simulink model "HIL_Testing_SW"  (Simulink 7.5)
settings: Solver=ode1  StartTime=0.0  StopTime=Inf  FixedStep=0.001  RelTol=1e-3
PostLoadFcn:
  | , if any(exist('dsrtsu_mdlpostloadfcn', 'file') == [2, 3, 6]), try dsrtsu_mdlpostloadfcn('Execute', bdroot); catch fprintf('Error in PostLoadFcn (dsrtsu_mdlpostloadfcn) for model "%s":\n %s\n', bdroot, lasterr); end, end,
undefined symbols (not defined in the file): CeBSER_Cnt_NumTempAxisPts, ChargeCord, ChargeCord_Control, ChargeToSOCCurr, ChrgCurrLim, CrntSens1Fine, CS_SOCSetPt, CyclerMaxChrgPwr, CyclerMaxDschrgPwr, deltaAhr, Drive_1, Drive_10, Drive_11, Drive_12, Drive_13, Drive_14, Drive_15, Drive_16, Drive_17, Drive_18, Drive_19, Drive_2, Drive_20, Drive_21, Drive_22, Drive_23, Drive_24, Drive_25, Drive_26, Drive_27, Drive_28, Drive_29, Drive_3, Drive_30, Drive_31, Drive_32, Drive_33, Drive_34, Drive_35, Drive_36, Drive_37, Drive_38, Drive_39, Drive_4, Drive_40, Drive_41, Drive_42, Drive_43, Drive_44, Drive_45, Drive_46, Drive_47, Drive_48, Drive_49, Drive_5, Drive_50, Drive_51, Drive_6, Drive_7, Drive_8 ... (+50)
libraries: simulink x129, rtican x50, rti2211sailib x5, rti2211serlib x5, rti2202miolib x3
(part 10 of 23)

== system HIL_Testing_SW/RX/Read EREV/Read PTEX ==
  Constant : Constant  Value=-1  OutDataType=fixdt(1, 16)  OutScaling=2^0
  PPEI_High_Vlt_Battery_Vlt_Status1 : rtican/RTICAN Receive (RX)   SystemSampleTime=-1  Reserved1=[]  Reserved2=[]  Reserved3=[]  Reserved4=[]  SfcnMessage=[]  Msg_Struct=[]  BoardTypeNo=[]  BoardNo=[]  ChannelNo=[]  Parameters=[]  DialogFcn=[]  UnitName=[]  Revision=[]  UnitValues=[]  DSProperties=struct('RTI',struct('Version',uint32(5),'BlockType',struct('isSLSource',uint8(1),'isSLSink',uint8(1),'isHWSource',uint8(0),'isHWSink',uint8(0),'isSetup',uint8(0),'isInline',uint8(1),'isNonInline',uint8(0),'isInterrupt',uint8(0),'isChannelwise',uint8(0)),'IOBoardType','RTICAN','UnitType','MESSAGE','Identifier','RX','DialogType','MSVC','BlockSet','RTICAN','SlaveProcessor','CAN'))  RTIBlockInterface=struct('OutputPortsWidth',int32([1 1 1 1 1 1 1 1]),'OutputPortsActive',[1 1 1 1 1 1 1 1],'OutputPortsName',{{'HVBatVltLwLmtCrnk','HVBatVltLwLmtCrnkV','HVBatVltLwLmt','HVBatVltLwLmtV','HVBatVltUpLmt','HVBatVltUpLmtV','HVBatPackPrcdVltg','HVBatPackPrcdVltgV'}},'OutputPortsDataType',{{'SS_DOUBLE','SS_DOUBLE','SS_DOUBLE','SS_DOUBLE','SS_DOUBLE','SS_DOUBLE','SS_DOUBLE','SS_DOUBLE'}},'OutputPortsLabel',{{'HVBatVltLwLmtCrnk','HVBatVltLwLmtCrnkV','HVBatVltLwLmt','HVBatVltLwLmtV','HVBatVltUpLmt','HVBatVltUpLmtV','HVBatPackPrcdVltg','HVBatPackPrcdVltgV'}},'OutputPortsLabelMode','ON','InputPortsWidth',int32(0),'InputPortsActive',0,'DialogFcn','rtican_message_interface_gui','BlockDisplay',{{'','center'}},'IconTransparency','on','ParameterTunableNames',{{}},'InitLevel',3,'BlockName',struct('Token',{{'PPEI_High_Vlt_Battery_Vlt_Status'}}),'SampleTime',{{-1}},'TriggerPort',{{'none'}},'EnablePort',{{'none'}})  RTIBlockParameters=struct('BoardTypeNo',{{4302,'OFF',[]}},'BoardNo',{{1,'ON',[1 16]}},'ChannelNo',{{2,'ON',[1 4]}},'Parameters',{{struct('DataFileSupport',struct('DataFileSelectedMaster',1,'DataFileSelectedLocal',1,'DataFileName',['c:\data\databases\8.4.5 (140425)\globala - pe.dbc|'],'DataFileDate',{{{['24-Apr-2014 15:33:48']}}},'SelectedFile',['..\databases\8.4.5 (140425)\globala - pe.dbc'],'InterfaceFcn','rtican_dbc_file_parser'),'Options',struct('StatusSelected',0,'TimeSelected',0,'DeltaTimeSelected',0,'BytePortSelected',0,'MessageLengthSelected',0,'TriggerPort',struct('Selected',0,'TriggerType',0),'UserCoding',struct('Selected',0,'InterfaceFile','UserDecodingFile','FcnName','UserDecodeFcn','InportSelected',0,'InportWidth',1,'OutportSelected',0,'OutportWidth',1),'EnablePortSelected',0,'SignalOnPortnameSelected',1,'UseRXService',0),'Message',struct('MsgOnBlocknameSelected',1,'MsgName','PPEI_High_Vlt_Battery_Vlt_Status','MsgIdFormat',0,'MsgId',983,'MsgLength',8,'NumSignals',8,'SampleTime',-1,'Signal',struct('SgnName',{'HVBatVltLwLmtCrnk','HVBatVltLwLmtCrnkV','HVBatVltLwLmt','HVBatVltLwLmtV','HVBatVltUpLmt','HVBatVltUpLmtV','HVBatPackPrcdVltg','HVBatPackPrcdVltgV'},'SgnStartBit',{0,10,16,26,32,42,48,58},'SgnLength',{10,1,10,1,10,1,10,1},'SgnType',{0,0,0,0,0,0,0,0},'ModeValue',{-1,-1,-1,-1,-1,-1,-1,-1},'DataType',{0,0,0,0,0,0,0,0},'ByteLayout',{2,2,2,2,2,2,2,2},'Factor',{0.52,1,0.52,1,0.52,1,0.52,1},'Offset',{0,0,0,0,0,0,0,0},'SgnComment',{{''},{''},{''},{''},{''},{''},{''},{''}},'SgnUnit',{'V','','V','','V','','V',''},'Min',{0,0,0,0,0,0,0,0},'Max',{531.96,1,531.96,1,531.96,1,531.96,1},'SLDataType',{'SS_DOUBLE','SS_DOUBLE','SS_DOUBLE','SS_DOUBLE','SS_DOUBLE','SS_DOUBLE','SS_DOUBLE','SS_DOUBLE'}),'MsgIdNumFormat',0,'MsgComment',{{''}}),'Version',1.2,'general',struct('isFromLib',0)),'OFF',[]}},'GroupId',{{struct('Group',{{'RTICAN'}},'No',5,'Behavior',{{'NAMECHANGE'}},'BlockType',{{'SINK'}},'NameChangeFlag',0),'OFF',[]}},'SFcnRTICANMessage',{{struct('MsgType','RX','SFcnPortType','Scalar','MsgName','PPEI_High_Vlt_Battery_Vlt_Status','MsgIdFormat','STD','MsgId',983,'MsgLength',8,'NumSignals',8,'SampleTime',-1,'Signal',struct('SgnName',{'HVBatVltLwLmtCrnk','HVBatVltLwLmtCrnkV','HVBatVltLwLmt','HVBatVltLwLmtV','HVBatVltUpLmt','HVBatVltUpLmtV','HVBatPackPrcdVltg','HVBatPackPrcdVltgV'},'SgnStartBit',{0,10,16,26,32,42,48,58},'SgnLength',{10,1,10,1,10,1,10,1},'SgnType',{'standard','standard','standard','standard','standard','standard','standard','standard'},'ModeValue',{-1,-1,-1,-1,-1,-1,-1,-1},'DataType',{['unsigned int'],['unsigned int'],['unsigned int'],['unsigned int'],['unsigned int'],['unsigned int'],['unsigned int'],['unsigned int']},'ByteLayout',{['motorola back.'],['motorola back.'],['motorola back.'],['motorola back.'],['motorola back.'],['motorola back.'],['motorola back.'],['motorola back.']},'Factor',{0.52,1,0.52,1,0.52,1,0.52,1},'Offset',{0,0,0,0,0,0,0,0},'SLDataType',{'SS_DOUBLE','SS_DOUBLE','SS_DOUBLE','SS_DOUBLE','SS_DOUBLE','SS_DOUBLE','SS_DOUBLE','SS_DOUBLE'}),'StatusSelected','no','TimeSelected','no','DeltaTimeSelected','no','BytePortSelected','no','MessageLengthSelected','no','TriggerPort',struct('Selected','no','TriggerType',0),'UserCoding',struct('Selected','no','InterfaceFile','UserDecodingFile','FcnName','UserDecodeFcn','InportSelected','no','InportWidth',1,'OutportSelected','no','OutportWidth',1),'EnablePortSelected','no','UseRXService','no','BoardType','DS4302','BoardNo',1,'ControllerNo',2),'OFF',[]}},'TLCFileName',{{'rtican_rx_message','OFF',[]}})  RTISFcnParameters=struct('SFcnRTICANMessage','struct','TLCFileName','char')  RTIBlockParaDefault=struct('BoardTypeNo',4302,'BoardNo',1,'ChannelNo',1,'Parameters',struct('DataFileSupport',struct('DataFileSelectedMaster',0,'DataFileSelectedLocal',0,'DataFileName','','DataFileDate','','SelectedFile',['<no file selected>']),'Options',struct('StatusSelected',1,'TimeSelected',1,'DeltaTimeSelected',1,'BytePortSelected',0,'MessageLengthSelected',0,'TriggerPort',struct('Selected',0,'TriggerType','rising'),'UserCoding',struct('Selected',0,'InterfaceFile','UserDecodingFile','FcnName','UserDecodeFcn','InportSelected',0,'InportWidth',1,'OutportSelected',0,'OutportWidth',1),'EnablePortSelected',0,'SignalOnPortnameSelected',1,'UseRXService',0),'Message',struct('MsgOnBlocknameSelected',0,'MsgName',['RX Message'],'MsgIdFormat',0,'MsgId',100,'MsgLength',8,'NumSignals',1,'SampleTime',-1,'Signal',struct('SgnName',['RX signal'],'SgnStartBit',0,'SgnLength',8,'SgnType',0,'ModeValue',-1,'DataType',0,'SLDataType','SS_DOUBLE','ByteLayout',0,'Factor',1,'Offset',0,'Min',0,'Max',255,'SgnComment',{{}},'SgnUnit',''),'MsgIdNumFormat',0,'MsgComment',{{''}}),'Version',1.2,'general',struct('isFromLib',1)),'GroupId',struct('Group',{{'RTICAN'}},'No',1,'Behavior',{{'NAMECHANGE'}},'BlockType',{{'SINK'}},'NameChangeFlag',0),'SFcnRTICANMessage',struct('MsgType','RX','MsgName',['RX Message'],'MsgIdFormat','STD','MsgId',100,'MsgLength',8,'NumSignals',1,'SampleTime',-1,'Signal',struct('SgnName',['RX signal'],'SgnStartBit',0,'SgnLength',8,'SgnType','standard','ModeValue',-1,'DataType',['unsigned int'],'ByteLayout',['little endian'],'SLDataType','SS_DOUBLE','Factor',1,'Offset',0),'StatusSelected','yes','TimeSelected','yes','DeltaTimeSelected','yes','BytePortSelected','no','MessageLengthSelected','no','EnablePortSelected','no','UserCoding',struct('Selected','no','InterfaceFile','UserDecodingFile','FcnName','UserDecodeFcn','InportSelected','no','InportWidth',1,'OutportSelected','no','OutportWidth',1),'TriggerPort',struct('Selected','no','TriggerType','rising'),'UseRXService','no','BoardType','DS4302','BoardNo',1,'ControllerNo',1,'SFcnPortType','Scalar'),'TLCFileName','rtican_rx_message')
      settings: AttributesFormatString=Group Id: RTICAN5\n
  PPEI_High_Volt_Batt_Current_Stat : rtican/RTICAN Receive (RX)   SystemSampleTime=-1  Reserved1=[]  Reserved2=[]  Reserved3=[]  Reserved4=[]  SfcnMessage=[]  Msg_Struct=[]  BoardTypeNo=[]  BoardNo=[]  ChannelNo=[]  Parameters=[]  DialogFcn=[]  UnitName=[]  Revision=[]  UnitValues=[]  DSProperties=struct('RTI',struct('Version',uint32(5),'BlockType',struct('isSLSource',uint8(1),'isSLSink',uint8(1),'isHWSource',uint8(0),'isHWSink',uint8(0),'isSetup',uint8(0),'isInline',uint8(1),'isNonInline',uint8(0),'isInterrupt',uint8(0),'isChannelwise',uint8(0)),'IOBoardType','RTICAN','UnitType','MESSAGE','Identifier','RX','DialogType','MSVC','BlockSet','RTICAN','SlaveProcessor','CAN'))  RTIBlockInterface=struct('OutputPortsWidth',int32([1 1 1 1 1 1]),'OutputPortsActive',[1 1 1 1 1 1],'OutputPortsName',{{'HVBatStOfChrgMin','HVBatCrntLwLmt','HVBatCrntLwLmtV','HVBatCrntUpLmt','HVBatCrntUpLmtV','HVBatSOCTrgtHiRes'}},'OutputPortsDataType',{{'SS_DOUBLE','SS_DOUBLE','SS_DOUBLE','SS_DOUBLE','SS_DOUBLE','SS_DOUBLE'}},'OutputPortsLabel',{{'HVBatStOfChrgMin','HVBatCrntLwLmt','HVBatCrntLwLmtV','HVBatCrntUpLmt','HVBatCrntUpLmtV','HVBatSOCTrgtHiRes'}},'OutputPortsLabelMode','ON','InputPortsWidth',int32(0),'InputPortsActive',0,'DialogFcn','rtican_message_interface_gui','BlockDisplay',{{'','center'}},'IconTransparency','on','ParameterTunableNames',{{}},'InitLevel',3,'BlockName',struct('Token',{{'PPEI_High_Volt_Batt_Current_Stat'}}),'SampleTime',{{-1}},'TriggerPort',{{'none'}},'EnablePort',{{'none'}})  RTIBlockParameters=struct('BoardTypeNo',{{4302,'OFF',[]}},'BoardNo',{{1,'ON',[1 16]}},'ChannelNo',{{2,'ON',[1 4]}},'Parameters',{{struct('DataFileSupport',struct('DataFileSelectedMaster',1,'DataFileSelectedLocal',1,'DataFileName',['c:\data\databases\8.4.5 (140425)\globala - pe.dbc|'],'DataFileDate',{{{['24-Apr-2014 15:33:48']}}},'SelectedFile',['..\databases\8.4.5 (140425)\globala - pe.dbc'],'InterfaceFcn','rtican_dbc_file_parser'),'Options',struct('StatusSelected',0,'TimeSelected',0,'DeltaTimeSelected',0,'BytePortSelected',0,'MessageLengthSelected',0,'TriggerPort',struct('Selected',0,'TriggerType',0),'UserCoding',struct('Selected',0,'InterfaceFile','UserDecodingFile','FcnName','UserDecodeFcn','InportSelected',0,'InportWidth',1,'OutportSelected',0,'OutportWidth',1),'EnablePortSelected',0,'SignalOnPortnameSelected',1,'UseRXService',0),'Message',struct('MsgOnBlocknameSelected',1,'MsgName','PPEI_High_Volt_Batt_Current_Stat','MsgIdFormat',0,'MsgId',981,'MsgLength',8,'NumSignals',6,'SampleTime',-1,'Signal',struct('SgnName',{'HVBatStOfChrgMin','HVBatCrntLwLmt','HVBatCrntLwLmtV','HVBatCrntUpLmt','HVBatCrntUpLmtV','HVBatSOCTrgtHiRes'},'SgnStartBit',{0,16,27,32,43,48},'SgnLength',{8,11,1,11,1,16},'SgnType',{0,0,0,0,0,0},'ModeValue',{-1,-1,-1,-1,-1,-1},'DataType',{0,0,0,0,0,0},'ByteLayout',{2,2,2,2,2,2},'Factor',{0.392157,0.3,1,0.3,1,0.001526},'Offset',{0,0,0,0,0,0},'SgnComment',{{''},{''},{''},{''},{''},{''}},'SgnUnit',{'','A','','A','','%'},'Min',{0,0,0,0,0,0},'Max',{100.000035,614.1,1,614.1,1,100},'SLDataType',{'SS_DOUBLE','SS_DOUBLE','SS_DOUBLE','SS_DOUBLE','SS_DOUBLE','SS_DOUBLE'}),'MsgIdNumFormat',0,'MsgComment',{{''}}),'Version',1.2,'general',struct('isFromLib',0)),'OFF',[]}},'GroupId',{{struct('Group',{{'RTICAN'}},'No',5,'Behavior',{{'NAMECHANGE'}},'BlockType',{{'SINK'}},'NameChangeFlag',0),'OFF',[]}},'SFcnRTICANMessage',{{struct('MsgType','RX','SFcnPortType','Scalar','MsgName','PPEI_High_Volt_Batt_Current_Stat','MsgIdFormat','STD','MsgId',981,'MsgLength',8,'NumSignals',6,'SampleTime',-1,'Signal',struct('SgnName',{'HVBatStOfChrgMin','HVBatCrntLwLmt','HVBatCrntLwLmtV','HVBatCrntUpLmt','HVBatCrntUpLmtV','HVBatSOCTrgtHiRes'},'SgnStartBit',{0,16,27,32,43,48},'SgnLength',{8,11,1,11,1,16},'SgnType',{'standard','standard','standard','standard','standard','standard'},'ModeValue',{-1,-1,-1,-1,-1,-1},'DataType',{['unsigned int'],['unsigned int'],['unsigned int'],['unsigned int'],['unsigned int'],['unsigned int']},'ByteLayout',{['motorola back.'],['motorola back.'],['motorola back.'],['motorola back.'],['motorola back.'],['motorola back.']},'Factor',{0.392157,0.3,1,0.3,1,0.001526},'Offset',{0,0,0,0,0,0},'SLDataType',{'SS_DOUBLE','SS_DOUBLE','SS_DOUBLE','SS_DOUBLE','SS_DOUBLE','SS_DOUBLE'}),'StatusSelected','no','TimeSelected','no','DeltaTimeSelected','no','BytePortSelected','no','MessageLengthSelected','no','TriggerPort',struct('Selected','no','TriggerType',0),'UserCoding',struct('Selected','no','InterfaceFile','UserDecodingFile','FcnName','UserDecodeFcn','InportSelected','no','InportWidth',1,'OutportSelected','no','OutportWidth',1),'EnablePortSelected','no','UseRXService','no','BoardType','DS4302','BoardNo',1,'ControllerNo',2),'OFF',[]}},'TLCFileName',{{'rtican_rx_message','OFF',[]}})  RTISFcnParameters=struct('SFcnRTICANMessage','struct','TLCFileName','char')  RTIBlockParaDefault=struct('BoardTypeNo',4302,'BoardNo',1,'ChannelNo',1,'Parameters',struct('DataFileSupport',struct('DataFileSelectedMaster',0,'DataFileSelectedLocal',0,'DataFileName','','DataFileDate','','SelectedFile',['<no file selected>']),'Options',struct('StatusSelected',1,'TimeSelected',1,'DeltaTimeSelected',1,'BytePortSelected',0,'MessageLengthSelected',0,'TriggerPort',struct('Selected',0,'TriggerType','rising'),'UserCoding',struct('Selected',0,'InterfaceFile','UserDecodingFile','FcnName','UserDecodeFcn','InportSelected',0,'InportWidth',1,'OutportSelected',0,'OutportWidth',1),'EnablePortSelected',0,'SignalOnPortnameSelected',1,'UseRXService',0),'Message',struct('MsgOnBlocknameSelected',0,'MsgName',['RX Message'],'MsgIdFormat',0,'MsgId',100,'MsgLength',8,'NumSignals',1,'SampleTime',-1,'Signal',struct('SgnName',['RX signal'],'SgnStartBit',0,'SgnLength',8,'SgnType',0,'ModeValue',-1,'DataType',0,'SLDataType','SS_DOUBLE','ByteLayout',0,'Factor',1,'Offset',0,'Min',0,'Max',255,'SgnComment',{{}},'SgnUnit',''),'MsgIdNumFormat',0,'MsgComment',{{''}}),'Version',1.2,'general',struct('isFromLib',1)),'GroupId',struct('Group',{{'RTICAN'}},'No',1,'Behavior',{{'NAMECHANGE'}},'BlockType',{{'SINK'}},'NameChangeFlag',0),'SFcnRTICANMessage',struct('MsgType','RX','MsgName',['RX Message'],'MsgIdFormat','STD','MsgId',100,'MsgLength',8,'NumSignals',1,'SampleTime',-1,'Signal',struct('SgnName',['RX signal'],'SgnStartBit',0,'SgnLength',8,'SgnType','standard','ModeValue',-1,'DataType',['unsigned int'],'ByteLayout',['little endian'],'SLDataType','SS_DOUBLE','Factor',1,'Offset',0),'StatusSelected','yes','TimeSelected','yes','DeltaTimeSelected','yes','BytePortSelected','no','MessageLengthSelected','no','EnablePortSelected','no','UserCoding',struct('Selected','no','InterfaceFile','UserDecodingFile','FcnName','UserDecodeFcn','InportSelected','no','InportWidth',1,'OutportSelected','no','OutportWidth',1),'TriggerPort',struct('Selected','no','TriggerType','rising'),'UseRXService','no','BoardType','DS4302','BoardNo',1,'ControllerNo',1,'SFcnPortType','Scalar'),'TLCFileName','rtican_rx_message')
      settings: AttributesFormatString=Group Id: RTICAN5\n
  PPEI_High_Volt_Batt_Dchrg_Pwrs1 : rtican/RTICAN Receive (RX)   SystemSampleTime=-1  Reserved1=[]  Reserved2=[]  Reserved3=[]  Reserved4=[]  SfcnMessage=[]  Msg_Struct=[]  BoardTypeNo=[]  BoardNo=[]  ChannelNo=[]  Parameters=[]  DialogFcn=[]  UnitName=[]  Revision=[]  UnitValues=[]  DSProperties=struct('RTI',struct('Version',uint32(5),'BlockType',struct('isSLSource',uint8(1),'isSLSink',uint8(1),'isHWSource',uint8(0),'isHWSink',uint8(0),'isSetup',uint8(0),'isInline',uint8(1),'isNonInline',uint8(0),'isInterrupt',uint8(0),'isChannelwise',uint8(0)),'IOBoardType','RTICAN','UnitType','MESSAGE','Identifier','RX','DialogType','MSVC','BlockSet','RTICAN','SlaveProcessor','CAN'))  RTIBlockInterface=struct('OutputPortsWidth',int32([1 1 1 1 1]),'OutputPortsActive',[1 1 1 1 1],'OutputPortsName',{{'HVBDP_ShrtTrmDischrgPwr','HVBDP_CrnkDischrgPwrV','HVBDP_Res','HVBDP_LngTrmDischrgPwr','HVBDP_CrnkDischrgPwr'}},'OutputPortsDataType',{{'SS_DOUBLE','SS_DOUBLE','SS_DOUBLE','SS_DOUBLE','SS_DOUBLE'}},'OutputPortsLabel',{{'HVBDP_ShrtTrmDischrgPwr','HVBDP_CrnkDischrgPwrV','HVBDP_Res','HVBDP_LngTrmDischrgPwr','HVBDP_CrnkDischrgPwr'}},'OutputPortsLabelMode','ON','InputPortsWidth',int32(0),'InputPortsActive',0,'DialogFcn','rtican_message_interface_gui','BlockDisplay',{{'','center'}},'IconTransparency','on','ParameterTunableNames',{{}},'InitLevel',3,'BlockName',struct('Token',{{'PPEI_High_Volt_Batt_Dchrg_Pwrs'}}),'SampleTime',{{-1}},'TriggerPort',{{'none'}},'EnablePort',{{'none'}})  RTIBlockParameters=struct('BoardTypeNo',{{4302,'OFF',[]}},'BoardNo',{{1,'ON',[1 16]}},'ChannelNo',{{2,'ON',[1 4]}},'Parameters',{{struct('DataFileSupport',struct('DataFileSelectedMaster',1,'DataFileSelectedLocal',1,'DataFileName',['c:\data\databases\8.0.1 (13015)\globala - pe.dbc|'],'DataFileDate',['24-Apr-2014 15:33:48'],'SelectedFile',['..\databases\8.4.5 (140425)\globala - pe.dbc'],'InterfaceFcn','rtican_dbc_file_parser'),'Options',struct('StatusSelected',0,'TimeSelected',0,'DeltaTimeSelected',0,'BytePortSelected',0,'MessageLengthSelected',0,'TriggerPort',struct('Selected',0,'TriggerType',0),'UserCoding',struct('Selected',0,'InterfaceFile','UserDecodingFile','FcnName','UserDecodeFcn','InportSelected',0,'InportWidth',1,'OutportSelected',0,'OutportWidth',1),'EnablePortSelected',0,'SignalOnPortnameSelected',1,'UseRXService',0),'Message',struct('MsgOnBlocknameSelected',1,'MsgName','PPEI_High_Volt_Batt_Dchrg_Pwrs','MsgIdFormat',0,'MsgId',987,'MsgLength',6,'NumSignals',5,'SampleTime',-1,'Signal',struct('SgnName',{'HVBDP_ShrtTrmDischrgPwr','HVBDP_CrnkDischrgPwrV','HVBDP_Res','HVBDP_LngTrmDischrgPwr','HVBDP_CrnkDischrgPwr'},'SgnStartBit',{13,24,25,26,37},'SgnLength',{11,1,1,11,11},'ByteLayout',{2,2,2,2,2},'Factor',{0.1,1,1,0.1,0.1},'Offset',{0,0,0,0,0},'SgnComment',{'','','','',''},'SgnUnit',{'kW','','','kW','kW'},'Min',{0,0,0,0,0},'Max',{204.7,1,1,204.7,204.7},'SgnType',{0,0,0,0,0},'SLDataType',{'SS_DOUBLE','SS_DOUBLE','SS_DOUBLE','SS_DOUBLE','SS_DOUBLE'},'DataType',{0,0,0,0,0},'ModeValue',{-1,-1,-1,-1,-1}),'MsgIdNumFormat',0,'MsgComment',{{''}}),'Version',1.2,'general',struct('isFromLib',0)),'OFF',[]}},'GroupId',{{struct('Group',{{'RTICAN'}},'No',5,'Behavior',{{'NAMECHANGE'}},'BlockType',{{'SINK'}},'NameChangeFlag',0),'OFF',[]}},'SFcnRTICANMessage',{{struct('MsgType','RX','SFcnPortType','Scalar','MsgName','PPEI_High_Volt_Batt_Dchrg_Pwrs','MsgIdFormat','STD','MsgId',987,'MsgLength',6,'NumSignals',5,'SampleTime',-1,'Signal',struct('SgnName',{'HVBDP_ShrtTrmDischrgPwr','HVBDP_CrnkDischrgPwrV','HVBDP_Res','HVBDP_LngTrmDischrgPwr','HVBDP_CrnkDischrgPwr'},'SgnStartBit',{13,24,25,26,37},'SgnLength',{11,1,1,11,11},'ByteLayout',{['motorola back.'],['motorola back.'],['motorola back.'],['motorola back.'],['motorola back.']},'Factor',{0.1,1,1,0.1,0.1},'Offset',{0,0,0,0,0},'SgnType',{'standard','standard','standard','standard','standard'},'SLDataType',{'SS_DOUBLE','SS_DOUBLE','SS_DOUBLE','SS_DOUBLE','SS_DOUBLE'},'DataType',{['unsigned int'],['unsigned int'],['unsigned int'],['unsigned int'],['unsigned int']},'ModeValue',{-1,-1,-1,-1,-1}),'StatusSelected','no','TimeSelected','no','DeltaTimeSelected','no','BytePortSelected','no','MessageLengthSelected','no','TriggerPort',struct('Selected','no','TriggerType',0),'UserCoding',struct('Selected','no','InterfaceFile','UserDecodingFile','FcnName','UserDecodeFcn','InportSelected','no','InportWidth',1,'OutportSelected','no','OutportWidth',1),'EnablePortSelected','no','UseRXService','no','BoardType','DS4302','BoardNo',1,'ControllerNo',2),'OFF',[]}},'TLCFileName',{{'rtican_rx_message','OFF',[]}})  RTISFcnParameters=struct('SFcnRTICANMessage','struct','TLCFileName','char')  RTIBlockParaDefault=struct('BoardTypeNo',4302,'BoardNo',1,'ChannelNo',1,'Parameters',struct('DataFileSupport',struct('DataFileSelectedMaster',0,'DataFileSelectedLocal',0,'DataFileName','','DataFileDate','','SelectedFile',['<no file selected>']),'Options',struct('StatusSelected',1,'TimeSelected',1,'DeltaTimeSelected',1,'BytePortSelected',0,'MessageLengthSelected',0,'TriggerPort',struct('Selected',0,'TriggerType','rising'),'UserCoding',struct('Selected',0,'InterfaceFile','UserDecodingFile','FcnName','UserDecodeFcn','InportSelected',0,'InportWidth',1,'OutportSelected',0,'OutportWidth',1),'EnablePortSelected',0,'SignalOnPortnameSelected',1,'UseRXService',0),'Message',struct('MsgOnBlocknameSelected',0,'MsgName',['RX Message'],'MsgIdFormat',0,'MsgId',100,'MsgLength',8,'NumSignals',1,'SampleTime',-1,'Signal',struct('SgnName',['RX signal'],'SgnStartBit',0,'SgnLength',8,'SgnType',0,'ModeValue',-1,'DataType',0,'SLDataType','SS_DOUBLE','ByteLayout',0,'Factor',1,'Offset',0,'Min',0,'Max',255,'SgnComment',{{}},'SgnUnit',''),'MsgIdNumFormat',0,'MsgComment',{{''}}),'Version',1.2,'general',struct('isFromLib',1)),'GroupId',struct('Group',{{'RTICAN'}},'No',1,'Behavior',{{'NAMECHANGE'}},'BlockType',{{'SINK'}},'NameChangeFlag',0),'SFcnRTICANMessage',struct('MsgType','RX','MsgName',['RX Message'],'MsgIdFormat','STD','MsgId',100,'MsgLength',8,'NumSignals',1,'SampleTime',-1,'Signal',struct('SgnName',['RX signal'],'SgnStartBit',0,'SgnLength',8,'SgnType','standard','ModeValue',-1,'DataType',['unsigned int'],'ByteLayout',['little endian'],'SLDataType','SS_DOUBLE','Factor',1,'Offset',0),'StatusSelected','yes','TimeSelected','yes','DeltaTimeSelected','yes','BytePortSelected','no','MessageLengthSelected','no','EnablePortSelected','no','UserCoding',struct('Selected','no','InterfaceFile','UserDecodingFile','FcnName','UserDecodeFcn','InportSelected','no','InportWidth',1,'OutportSelected','no','OutportWidth',1),'TriggerPort',struct('Selected','no','TriggerType','rising'),'UseRXService','no','BoardType','DS4302','BoardNo',1,'ControllerNo',1,'SFcnPortType','Scalar'),'TLCFileName','rtican_rx_message')
      settings: AttributesFormatString=Group Id: RTICAN5\n
  PPEI_High_Voltage_Batt_Chrg_Pwrs1 : rtican/RTICAN Receive (RX)   SystemSampleTime=-1  Reserved1=[]  Reserved2=[]  Reserved3=[]  Reserved4=[]  SfcnMessage=[]  Msg_Struct=[]  BoardTypeNo=[]  BoardNo=[]  ChannelNo=[]  Parameters=[]  DialogFcn=[]  UnitName=[]  Revision=[]  UnitValues=[]  DSProperties=struct('RTI',struct('Version',uint32(5),'BlockType',struct('isSLSource',uint8(1),'isSLSink',uint8(1),'isHWSource',uint8(0),'isHWSink',uint8(0),'isSetup',uint8(0),'isInline',uint8(1),'isNonInline',uint8(0),'isInterrupt',uint8(0),'isChannelwise',uint8(0)),'IOBoardType','RTICAN','UnitType','MESSAGE','Identifier','RX','DialogType','MSVC','BlockSet','RTICAN','SlaveProcessor','CAN'))  RTIBlockInterface=struct('OutputPortsWidth',int32([1 1 1 1 1 1 1 1]),'OutputPortsActive',[1 1 1 1 1 1 1 1],'OutputPortsName',{{'HVBatSOCHiRes','HVBatOutOfEnrgyStat','HVBatSOCHiResV','HVBCP_ShrtTrmChrgPwr','HVBCP_CrnkChrgPwrV','HVBCP_Res','HVBCP_LngTrmChrgPwr','HVBCP_CrnkChrgPwr'}},'OutputPortsDataType',{{'SS_DOUBLE','SS_DOUBLE','SS_DOUBLE','SS_DOUBLE','SS_DOUBLE','SS_DOUBLE','SS_DOUBLE','SS_DOUBLE'}},'OutputPortsLabel',{{'HVBatSOCHiRes','HVBatOutOfEnrgyStat','HVBatSOCHiResV','HVBCP_ShrtTrmChrgPwr','HVBCP_CrnkChrgPwrV','HVBCP_Res','HVBCP_LngTrmChrgPwr','HVBCP_CrnkChrgPwr'}},'OutputPortsLabelMode','ON','InputPortsWidth',int32(0),'InputPortsActive',0,'DialogFcn','rtican_message_interface_gui','BlockDisplay',{{'','center'}},'IconTransparency','on','ParameterTunableNames',{{}},'InitLevel',3,'BlockName',struct('Token',{{'PPEI_High_Voltage_Batt_Chrg_Pwrs'}}),'SampleTime',{{-1}},'TriggerPort',{{'none'}},'EnablePort',{{'none'}})  RTIBlockParameters=struct('BoardTypeNo',{{4302,'OFF',[]}},'BoardNo',{{1,'ON',[1 16]}},'ChannelNo',{{2,'ON',[1 4]}},'Parameters',{{struct('DataFileSupport',struct('DataFileSelectedMaster',1,'DataFileSelectedLocal',1,'DataFileName',['c:\data\databases\8.0.1 (13015)\globala - pe.dbc|'],'DataFileDate',['24-Apr-2014 15:33:48'],'SelectedFile',['..\databases\8.4.5 (140425)\globala - pe.dbc'],'InterfaceFcn','rtican_dbc_file_parser'),'Options',struct('StatusSelected',0,'TimeSelected',0,'DeltaTimeSelected',0,'BytePortSelected',0,'MessageLengthSelected',0,'TriggerPort',struct('Selected',0,'TriggerType',0),'UserCoding',struct('Selected',0,'InterfaceFile','UserDecodingFile','FcnName','UserDecodeFcn','InportSelected',0,'InportWidth',1,'OutportSelected',0,'OutportWidth',1),'EnablePortSelected',0,'SignalOnPortnameSelected',1,'UseRXService',0),'Message',struct('MsgOnBlocknameSelected',1,'MsgName','PPEI_High_Voltage_Batt_Chrg_Pwrs','MsgIdFormat',0,'MsgId',986,'MsgLength',8,'NumSignals',8,'SampleTime',-1,'Signal',struct('SgnName',{'HVBatSOCHiRes','HVBatOutOfEnrgyStat','HVBatSOCHiResV','HVBCP_ShrtTrmChrgPwr','HVBCP_CrnkChrgPwrV','HVBCP_Res','HVBCP_LngTrmChrgPwr','HVBCP_CrnkChrgPwr'},'SgnStartBit',{0,25,28,29,40,41,42,53},'SgnLength',{16,3,1,11,1,1,11,11},'ByteLayout',{2,2,2,2,2,2,2,2},'Factor',{0.00152593,1,1,0.1,1,1,0.1,0.1},'Offset',{0,0,0,0,0,0,0,0},'SgnComment',{'','','','','','','',''},'SgnUnit',{'%','','','kW','','','kW','kW'},'Min',{0,0,0,0,0,0,0,0},'Max',{100.00182255,7,1,204.7,1,1,204.7,204.7},'SgnType',{0,0,0,0,0,0,0,0},'SLDataType',{'SS_DOUBLE','SS_DOUBLE','SS_DOUBLE','SS_DOUBLE','SS_DOUBLE','SS_DOUBLE','SS_DOUBLE','SS_DOUBLE'},'DataType',{0,0,0,0,0,0,0,0},'ModeValue',{-1,-1,-1,-1,-1,-1,-1,-1}),'MsgIdNumFormat',0,'MsgComment',{{''}}),'Version',1.2,'general',struct('isFromLib',0)),'OFF',[]}},'GroupId',{{struct('Group',{{'RTICAN'}},'No',5,'Behavior',{{'NAMECHANGE'}},'BlockType',{{'SINK'}},'NameChangeFlag',0),'OFF',[]}},'SFcnRTICANMessage',{{struct('MsgType','RX','SFcnPortType','Scalar','MsgName','PPEI_High_Voltage_Batt_Chrg_Pwrs','MsgIdFormat','STD','MsgId',986,'MsgLength',8,'NumSignals',8,'SampleTime',-1,'Signal',struct('SgnName',{'HVBatSOCHiRes','HVBatOutOfEnrgyStat','HVBatSOCHiResV','HVBCP_ShrtTrmChrgPwr','HVBCP_CrnkChrgPwrV','HVBCP_Res','HVBCP_LngTrmChrgPwr','HVBCP_CrnkChrgPwr'},'SgnStartBit',{0,25,28,29,40,41,42,53},'SgnLength',{16,3,1,11,1,1,11,11},'ByteLayout',{['motorola back.'],['motorola back.'],['motorola back.'],['motorola back.'],['motorola back.'],['motorola back.'],['motorola back.'],['motorola back.']},'Factor',{0.00152593,1,1,0.1,1,1,0.1,0.1},'Offset',{0,0,0,0,0,0,0,0},'SgnType',{'standard','standard','standard','standard','standard','standard','standard','standard'},'SLDataType',{'SS_DOUBLE','SS_DOUBLE','SS_DOUBLE','SS_DOUBLE','SS_DOUBLE','SS_DOUBLE','SS_DOUBLE','SS_DOUBLE'},'DataType',{['unsigned int'],['unsigned int'],['unsigned int'],['unsigned int'],['unsigned int'],['unsigned int'],['unsigned int'],['unsigned int']},'ModeValue',{-1,-1,-1,-1,-1,-1,-1,-1}),'StatusSelected','no','TimeSelected','no','DeltaTimeSelected','no','BytePortSelected','no','MessageLengthSelected','no','TriggerPort',struct('Selected','no','TriggerType',0),'UserCoding',struct('Selected','no','InterfaceFile','UserDecodingFile','FcnName','UserDecodeFcn','InportSelected','no','InportWidth',1,'OutportSelected','no','OutportWidth',1),'EnablePortSelected','no','UseRXService','no','BoardType','DS4302','BoardNo',1,'ControllerNo',2),'OFF',[]}},'TLCFileName',{{'rtican_rx_message','OFF',[]}})  RTISFcnParameters=struct('SFcnRTICANMessage','struct','TLCFileName','char')  RTIBlockParaDefault=struct('BoardTypeNo',4302,'BoardNo',1,'ChannelNo',1,'Parameters',struct('DataFileSupport',struct('DataFileSelectedMaster',0,'DataFileSelectedLocal',0,'DataFileName','','DataFileDate','','SelectedFile',['<no file selected>']),'Options',struct('StatusSelected',1,'TimeSelected',1,'DeltaTimeSelected',1,'BytePortSelected',0,'MessageLengthSelected',0,'TriggerPort',struct('Selected',0,'TriggerType','rising'),'UserCoding',struct('Selected',0,'InterfaceFile','UserDecodingFile','FcnName','UserDecodeFcn','InportSelected',0,'InportWidth',1,'OutportSelected',0,'OutportWidth',1),'EnablePortSelected',0,'SignalOnPortnameSelected',1,'UseRXService',0),'Message',struct('MsgOnBlocknameSelected',0,'MsgName',['RX Message'],'MsgIdFormat',0,'MsgId',100,'MsgLength',8,'NumSignals',1,'SampleTime',-1,'Signal',struct('SgnName',['RX signal'],'SgnStartBit',0,'SgnLength',8,'SgnType',0,'ModeValue',-1,'DataType',0,'SLDataType','SS_DOUBLE','ByteLayout',0,'Factor',1,'Offset',0,'Min',0,'Max',255,'SgnComment',{{}},'SgnUnit',''),'MsgIdNumFormat',0,'MsgComment',{{''}}),'Version',1.2,'general',struct('isFromLib',1)),'GroupId',struct('Group',{{'RTICAN'}},'No',1,'Behavior',{{'NAMECHANGE'}},'BlockType',{{'SINK'}},'NameChangeFlag',0),'SFcnRTICANMessage',struct('MsgType','RX','MsgName',['RX Message'],'MsgIdFormat','STD','MsgId',100,'MsgLength',8,'NumSignals',1,'SampleTime',-1,'Signal',struct('SgnName',['RX signal'],'SgnStartBit',0,'SgnLength',8,'SgnType','standard','ModeValue',-1,'DataType',['unsigned int'],'ByteLayout',['little endian'],'SLDataType','SS_DOUBLE','Factor',1,'Offset',0),'StatusSelected','yes','TimeSelected','yes','DeltaTimeSelected','yes','BytePortSelected','no','MessageLengthSelected','no','EnablePortSelected','no','UserCoding',struct('Selected','no','InterfaceFile','UserDecodingFile','FcnName','UserDecodeFcn','InportSelected','no','InportWidth',1,'OutportSelected','no','OutportWidth',1),'TriggerPort',struct('Selected','no','TriggerType','rising'),'UseRXService','no','BoardType','DS4302','BoardNo',1,'ControllerNo',1,'SFcnPortType','Scalar'),'TLCFileName','rtican_rx_message')
      settings: AttributesFormatString=Group Id: RTICAN5\n
  Product : Product  OutDataType=fixdt(1, 16)  OutScaling=2^0  RndMeth=Zero
  Terminator{,1..20} (21 alike) : Terminator
  LT_PwrDschLmt : Outport  OutDataType=sfix(16)  OutScaling=2^0
  LT_PwrChgLmt : Outport  Port=2  OutDataType=sfix(16)  OutScaling=2^0
  SOC : Outport  Port=3  OutDataType=sfix(16)  OutScaling=2^0
  HVBatVltUpLmt_CAN : Outport  Port=4  OutDataType=sfix(16)  OutScaling=2^0
  HVBatVltLwLmt_CAN : Outport  Port=5  OutDataType=sfix(16)  OutScaling=2^0
  HVBatStOfChrgMin_CAN : Outport  Port=6  OutDataType=sfix(16)  OutScaling=2^0
  HVBatCrntLwLmt_CAN : Outport  Port=7  OutDataType=sfix(16)  OutScaling=2^0
  HVBatCrntUpLmt_CAN : Outport  Port=8  OutDataType=sfix(16)  OutScaling=2^0
  wires:
  PPEI_High_Volt_Batt_Dchrg_Pwrs1/1 -> Terminator/1  "HVBDP_ShrtTrmDischrgPwr"
  PPEI_High_Volt_Batt_Dchrg_Pwrs1/2 -> Terminator2/1  "HVBDP_CrnkDischrgPwrV"
  PPEI_High_Volt_Batt_Dchrg_Pwrs1/3 -> Terminator3/1  "HVBDP_Res"
  PPEI_High_Volt_Batt_Dchrg_Pwrs1/4 -> LT_PwrDschLmt/1  "HVBDP_LngTrmDischrgPwr"
  PPEI_High_Volt_Batt_Dchrg_Pwrs1/5 -> Terminator6/1  "HVBDP_CrnkDischrgPwr"
  PPEI_High_Voltage_Batt_Chrg_Pwrs1/1 -> SOC/1  "HVBatSOCHiRes"
  PPEI_High_Voltage_Batt_Chrg_Pwrs1/2 -> Terminator7/1  "HVBatOutOfEnrgyStat"
  PPEI_High_Voltage_Batt_Chrg_Pwrs1/3 -> Terminator8/1  "HVBatSOCHiResV"
  PPEI_High_Voltage_Batt_Chrg_Pwrs1/4 -> Terminator9/1  "HVBCP_ShrtTrmChrgPwr"
  PPEI_High_Voltage_Batt_Chrg_Pwrs1/5 -> Terminator10/1  "HVBCP_CrnkChrgPwrV"
  PPEI_High_Voltage_Batt_Chrg_Pwrs1/6 -> Terminator11/1  "HVBCP_Res"
  PPEI_High_Voltage_Batt_Chrg_Pwrs1/8 -> Terminator12/1  "HVBCP_CrnkChrgPwr"
  PPEI_High_Voltage_Batt_Chrg_Pwrs1/7 -> LT_PwrChgLmt/1  "HVBCP_LngTrmChrgPwr"
  PPEI_High_Vlt_Battery_Vlt_Status1/1 -> Terminator5/1  "HVBatVltLwLmtCrnk"
  PPEI_High_Vlt_Battery_Vlt_Status1/5 -> HVBatVltUpLmt_CAN/1  "HVBatVltUpLmt"
  PPEI_High_Vlt_Battery_Vlt_Status1/2 -> Terminator13/1  "HVBatVltLwLmtCrnkV"
  PPEI_High_Vlt_Battery_Vlt_Status1/3 -> HVBatVltLwLmt_CAN/1  "HVBatVltLwLmt"
  PPEI_High_Vlt_Battery_Vlt_Status1/4 -> Terminator14/1  "HVBatVltLwLmtV"
  PPEI_High_Vlt_Battery_Vlt_Status1/6 -> Terminator15/1  "HVBatVltUpLmtV"
  PPEI_High_Vlt_Battery_Vlt_Status1/7 -> Terminator16/1  "HVBatPackPrcdVltg"
  PPEI_High_Vlt_Battery_Vlt_Status1/8 -> Terminator17/1  "HVBatPackPrcdVltgV"
  PPEI_High_Volt_Batt_Current_Stat/1 -> HVBatStOfChrgMin_CAN/1  "HVBatStOfChrgMin"
  PPEI_High_Volt_Batt_Current_Stat/3 -> Terminator19/1  "HVBatCrntLwLmtV"
  PPEI_High_Volt_Batt_Current_Stat/4 -> HVBatCrntUpLmt_CAN/1  "HVBatCrntUpLmt"
  PPEI_High_Volt_Batt_Current_Stat/5 -> Terminator20/1  "HVBatCrntUpLmtV"
  Constant/1 -> Product/2
  PPEI_High_Volt_Batt_Current_Stat/2 -> Product/1  "HVBatCrntLwLmt"
  Product/1 -> HVBatCrntLwLmt_CAN/1

== system HIL_Testing_SW/TX/Chamber/ChamberT_SwitchSlct ==
  BatTemp : Inport  OutDataType=fixdt(1, 16)  OutScaling=2^0
  SetChamberT_ToBatTemp : Inport  Port=2  OutDataType=fixdt(1, 16)  OutScaling=2^0
  Trigger : TriggerPort  TriggerType=function-call
  ChamberTempSwitchSelect : Lookup  InputValues=[-30,-27.5,-25,-22.5,-20,-17.5,-15,-12.5,-10,-7.5,-5,-2.5,0,2.5,5,7.5,10,12.5,15,17.5,20,22.5,25,27.5,30,32.5,35,37.5,40,42.5,45,47.5,50,52.5,55,57.5,60,62.5,65]  Table=uint8([1,2,3,4,5,6,7,8,9,10,11,12,13,14,15,16,17,18,19,20,21,22,23,24,25,26,27,28,29,30,31,32,33,34,35,36,37,38,39]);  LookUpMeth=Use Input Nearest  OutDataTypeMode=uint8  OutDataType=fixdt(1, 16)  OutScaling=2^0  OutDataTypeStr=uint8  RndMeth=Nearest
  ManualChamberT_SP : Constant  Value=single(25)  OutDataType=fixdt(1, 16)  OutScaling=2^0
  Switch : Switch  Threshold=.5  OutDataType=fixdt(1, 16)  OutScaling=2^0
  BatT_SwitchNumSlct : Outport  OutDataType=sfix(16)  OutScaling=2^0
  wires:
  ChamberTempSwitchSelect/1 -> BatT_SwitchNumSlct/1  "BatT_SwitchNumSlct"
  SetChamberT_ToBatTemp/1 -> Switch/2
  Switch/1 -> ChamberTempSwitchSelect/1
  BatTemp/1 -> Switch/1
  ManualChamberT_SP/1 -> Switch/3

== system HIL_Testing_SW/TX/Chamber/SendTxToChamber ==
  ChamberTempCommand : Inport  OutDataType=fixdt(1, 16)  OutScaling=2^0
  Trigger : TriggerPort  TriggerType=function-call
  ChamberSend8Bytes : Constant  Value=8  OutDataTypeMode=uint32  OutDataType=fixdt(1, 16)  OutScaling=2^0  OutDataTypeStr=uint32
  ChamberSendNoBytes : Constant  Value=0  OutDataTypeMode=uint32  OutDataType=fixdt(1, 16)  OutScaling=2^0  OutDataTypeStr=uint32
  DS2211SER_TX_B1 : rti2211serlib/DS2211SER_TX_B1  SystemSampleTime=-1  Reserved1=[]  Reserved2=[]  Reserved3=[]  Reserved4=[]  DSProperties=struct('RTI',struct('IOBoardType',{{'DS2211','SER'}},'SlaveProcessor','NONE','Version',uint32(1),'BlockType',struct('isSLSource',uint8(1),'isSLSink',uint8(1),'isHWSource',uint8(1),'isHWSink',uint8(0),'isSetup',uint8(0),'isInline',uint8(1),'isNonInline',uint8(0),'isInterrupt',uint8(0),'isChannelwise',uint8(1)),'UnitType','GENSER','Identifier','TRANSMIT','DialogType','ML','BlockSet','NONE'))  RTIBlockInterface=struct('BlockName',struct('Token',{{'DS2211SER_TX_B'}},'BlockParam',{{'BoardNo'}}),'InputPortsWidth',int32([8 1]),'InputPortsActive',[1 1],'InputPortsDataType',{{'SS_UINT8','SS_UINT32'}},'InputPortsName',{{'TXBytes','NumBytes'}},'OutputPortsWidth',int32([1 1]),'OutputPortsActive',[1 1],'OutputPortsDataType',{{'SS_UINT32','SS_INT32'}},'OutputPortsName',{{'NumTXBytes','Status'}},'BlockDisplay',{{['Serial Transmit'],'center'}},'IconTransparency','on','ParameterTunableNames',{{'BytesRefNumOf'}},'InitLevel',2,'DialogFcn','guigensertransmit','MaskDescription',['To write data to the UART SW FIFO.'])  RTIBlockParameters=struct('BoardNo',{{1,'ON',[1 16]}},'ChannelNo',{{1,'ON',[1 1]}},'ChannelNumOf',{{1,'OFF',[]}},'TransmitFifoOverrunMode',{{1,'OFF',[]}},'ParamTunableMode',{{1,'OFF',[]}},'BytesRefNumOfT',{{'1','OFF',[1 inf]}},'BytesRefNumOfNT',{{'1','OFF',[1 inf]}},'BytesRefNumOfMax',{{'8','OFF',[1 inf]}},'BytesRefNumOfMode',{{0,'OFF',[]}},'BytesActNumOfMode',{{1,'OFF',[]}},'TransmissionStatusMode',{{1,'OFF',[]}},'FifoSizeDefault',{{64,'OFF',[]}},'TLCFileName',{{'rtigensertransmit','OFF',[]}})  RTISFcnParameters=struct('BoardNo','double','ChannelNo','double','ChannelNumOf','double','TransmitFifoOverrunMode','double','ParamTunableMode','double','BytesRefNumOfT','double','BytesRefNumOfNT','double','BytesRefNumOfMax','double','BytesRefNumOfMode','double','BytesActNumOfMode','double','TransmissionStatusMode','double','TLCFileName','char')  RTIBlockParaDefault=struct('BoardNo',1,'ChannelNo',1,'ChannelNumOf',1,'TransmitFifoOverrunMode',1,'ParamTunableMode',1,'BytesRefNumOfT',1,'BytesRefNumOfNT',1,'BytesRefNumOfMax',1,'BytesRefNumOfMode',0,'BytesActNumOfMode',1,'TransmissionStatusMode',1,'FifoSizeDefault',64,'TLCFileName','rtigensertransmit')
  SendNothingToChamber : Constant  Value=[0 0 0 0 0 0 0 0]  OutDataTypeMode=uint8  OutDataType=fixdt(1, 16)  OutScaling=2^0  OutDataTypeStr=uint8
  Switch : Switch  OutDataType=fixdt(1, 16)  OutScaling=2^0
  Switch1 : Switch  OutDataType=fixdt(1, 16)  OutScaling=2^0
  Terminator : Terminator
  Terminator1 : Terminator
  dSPACEControlsChamberTemp : Constant  Value=0  OutDataTypeMode=boolean  OutDataType=fixdt(1, 16)  OutScaling=2^0  OutDataTypeStr=boolean
  wires:
  DS2211SER_TX_B1/2 -> Terminator1/1
  SendNothingToChamber/1 -> Switch/3
  ChamberTempCommand/1 -> Switch/1
  dSPACEControlsChamberTemp/1 -> Switch/2, Switch1/2
  Switch/1 -> DS2211SER_TX_B1/1  "ChamberTempCommand"
  DS2211SER_TX_B1/1 -> Terminator/1
  ChamberSendNoBytes/1 -> Switch1/3
  ChamberSend8Bytes/1 -> Switch1/1
  Switch1/1 -> DS2211SER_TX_B1/2  "ChamberNumBytes"

== system HIL_Testing_SW/TX/Chamber/Trigger_200ms ==
  Function-Call Generator : simulink/Ports & Subsystems/Function-Call Generator  sample_time=.4  numberOfIterations=1
  Output Parameter : Outport  OutDataType=sfix(16)  OutScaling=2^0
  wires:
  Function-Call Generator/1 -> Output Parameter/1

== system HIL_Testing_SW/TX/Chamber/Trigger_200ms2 ==
  Function-Call Generator : simulink/Ports & Subsystems/Function-Call Generator  sample_time=.2  numberOfIterations=1
  Output Parameter : Outport  OutDataType=sfix(16)  OutScaling=2^0
  wires:
  Function-Call Generator/1 -> Output Parameter/1

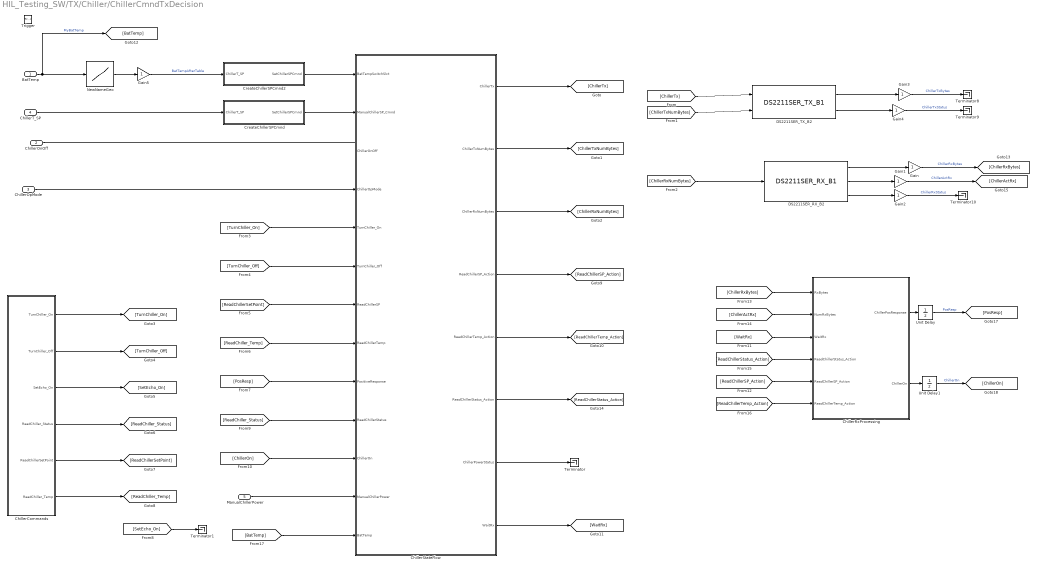
== system HIL_Testing_SW/TX/Chiller/ChillerCmndTxDecision ==
  BatTemp : Inport  OutDataType=fixdt(1, 16)  OutScaling=2^0
  ChillerOnOff : Inport  Port=2  OutDataType=fixdt(1, 16)  OutScaling=2^0
  ChillerOpMode : Inport  Port=3  OutDataType=fixdt(1, 16)  OutScaling=2^0
  ChillerT_SP : Inport  Port=4  OutDataType=fixdt(1, 16)  OutScaling=2^0
  ManualChillerPower : Inport  Port=5  OutDataType=fixdt(1, 16)  OutScaling=2^0
  Trigger : TriggerPort  TriggerType=function-call
  ChillerCommands : Subsystem
  ChillerRxProcessing : Subsystem
  ChillerStateFlow : Stateflow chart  TreatAsAtomicUnit=on
  CreateChillerSPCmnd : Subsystem
  CreateChillerSPCmnd2 : Subsystem
  DS2211SER_RX_B2 : rti2211serlib/DS2211SER_RX_B1  SystemSampleTime=-1  Reserved1=[]  Reserved2=[]  Reserved3=[]  Reserved4=[]  DSProperties=struct('RTI',struct('IOBoardType',{{'DS2211','SER'}},'SlaveProcessor','NONE','Version',uint32(1),'BlockType',struct('isSLSource',uint8(1),'isSLSink',uint8(1),'isHWSource',uint8(0),'isHWSink',uint8(1),'isSetup',uint8(0),'isInline',uint8(1),'isNonInline',uint8(0),'isInterrupt',uint8(0),'isChannelwise',uint8(1)),'UnitType','GENSER','Identifier','RECEIVE','DialogType','ML','BlockSet','NONE'))  RTIBlockInterface=struct('BlockName',struct('Token',{{'DS2211SER_RX_B'}},'BlockParam',{{'BoardNo'}}),'InputPortsWidth',int32(1),'InputPortsActive',1,'InputPortsDataType',{{'SS_UINT32'}},'InputPortsName',{{'NumBytes'}},'OutputPortsWidth',int32([7 1 1]),'OutputPortsActive',[1 1 1],'OutputPortsDataType',{{'SS_UINT8','SS_UINT32','SS_INT32'}},'OutputPortsName',{{'RXBytes','NumRXBytes','Status'}},'BlockDisplay',{{['Serial Receive'],'center'}},'IconTransparency','on','ParameterTunableNames',{{'BytesRefNumOf'}},'InitLevel',2,'DialogFcn','guigenserreceive','MaskDescription',['To read data from the UART SW FIFO.'])  RTIBlockParameters=struct('BoardNo',{{2,'ON',[1 16]}},'ChannelNo',{{1,'ON',[1 1]}},'ChannelNumOf',{{1,'OFF',[]}},'ReceptionDataMode',{{1,'OFF',[]}},'ParamTunableMode',{{1,'OFF',[]}},'BytesRefNumOfT',{{'7','OFF',[1 inf]}},'BytesRefNumOfNT',{{'7','OFF',[1 inf]}},'BytesRefNumOfMax',{{'7','OFF',[1 inf]}},'BytesRefNumOfMode',{{0,'OFF',[]}},'BytesActNumOfMode',{{1,'OFF',[]}},'ReceptionStatusMode',{{1,'OFF',[]}},'FifoSizeDefault',{{64,'OFF',[]}},'TLCFileName',{{'rtigenserreceive','OFF',[]}})  RTISFcnParameters=struct('BoardNo','double','ChannelNo','double','ChannelNumOf','double','ReceptionDataMode','double','ParamTunableMode','double','BytesRefNumOfT','double','BytesRefNumOfNT','double','BytesRefNumOfMax','double','BytesRefNumOfMode','double','BytesActNumOfMode','double','ReceptionStatusMode','double','TLCFileName','char')  RTIBlockParaDefault=struct('BoardNo',1,'ChannelNo',1,'ChannelNumOf',1,'ReceptionDataMode',1,'ParamTunableMode',1,'BytesRefNumOfT',1,'BytesRefNumOfNT',1,'BytesRefNumOfMax',1,'BytesRefNumOfMode',0,'BytesActNumOfMode',1,'ReceptionStatusMode',1,'FifoSizeDefault',64,'TLCFileName','rtigenserreceive')
  DS2211SER_TX_B2 : rti2211serlib/DS2211SER_TX_B1  SystemSampleTime=-1  Reserved1=[]  Reserved2=[]  Reserved3=[]  Reserved4=[]  DSProperties=struct('RTI',struct('IOBoardType',{{'DS2211','SER'}},'SlaveProcessor','NONE','Version',uint32(1),'BlockType',struct('isSLSource',uint8(1),'isSLSink',uint8(1),'isHWSource',uint8(1),'isHWSink',uint8(0),'isSetup',uint8(0),'isInline',uint8(1),'isNonInline',uint8(0),'isInterrupt',uint8(0),'isChannelwise',uint8(1)),'UnitType','GENSER','Identifier','TRANSMIT','DialogType','ML','BlockSet','NONE'))  RTIBlockInterface=struct('BlockName',struct('Token',{{'DS2211SER_TX_B'}},'BlockParam',{{'BoardNo'}}),'InputPortsWidth',int32([8 1]),'InputPortsActive',[1 1],'InputPortsDataType',{{'SS_UINT8','SS_UINT32'}},'InputPortsName',{{'TXBytes','NumBytes'}},'OutputPortsWidth',int32([1 1]),'OutputPortsActive',[1 1],'OutputPortsDataType',{{'SS_UINT32','SS_INT32'}},'OutputPortsName',{{'NumTXBytes','Status'}},'BlockDisplay',{{['Serial Transmit'],'center'}},'IconTransparency','on','ParameterTunableNames',{{'BytesRefNumOf'}},'InitLevel',2,'DialogFcn','guigensertransmit','MaskDescription',['To write data to the UART SW FIFO.'])  RTIBlockParameters=struct('BoardNo',{{2,'ON',[1 16]}},'ChannelNo',{{1,'ON',[1 1]}},'ChannelNumOf',{{1,'OFF',[]}},'TransmitFifoOverrunMode',{{1,'OFF',[]}},'ParamTunableMode',{{1,'OFF',[]}},'BytesRefNumOfT',{{'1','OFF',[1 inf]}},'BytesRefNumOfNT',{{'1','OFF',[1 inf]}},'BytesRefNumOfMax',{{'8','OFF',[1 inf]}},'BytesRefNumOfMode',{{0,'OFF',[]}},'BytesActNumOfMode',{{1,'OFF',[]}},'TransmissionStatusMode',{{1,'OFF',[]}},'FifoSizeDefault',{{64,'OFF',[]}},'TLCFileName',{{'rtigensertransmit','OFF',[]}})  RTISFcnParameters=struct('BoardNo','double','ChannelNo','double','ChannelNumOf','double','TransmitFifoOverrunMode','double','ParamTunableMode','double','BytesRefNumOfT','double','BytesRefNumOfNT','double','BytesRefNumOfMax','double','BytesRefNumOfMode','double','BytesActNumOfMode','double','TransmissionStatusMode','double','TLCFileName','char')  RTIBlockParaDefault=struct('BoardNo',1,'ChannelNo',1,'ChannelNumOf',1,'TransmitFifoOverrunMode',1,'ParamTunableMode',1,'BytesRefNumOfT',1,'BytesRefNumOfNT',1,'BytesRefNumOfMax',1,'BytesRefNumOfMode',0,'BytesActNumOfMode',1,'TransmissionStatusMode',1,'FifoSizeDefault',64,'TLCFileName','rtigensertransmit')
  Gain{,1..4} (5 alike) : Gain  ParameterDataType=fixdt(1, 16)  ParameterScaling=2^0  OutDataType=fixdt(1, 16)  OutScaling=2^0
  Gain5 : Gain  ParameterDataType=fixdt(1, 16)  ParameterScaling=2^0  OutDataTypeMode=single  OutDataType=fixdt(1, 16)  OutScaling=2^0  OutDataTypeStr=single
  NewNameGeo : Lookup  InputValues=[-30,-20,-10,-9,-8,-7,-6,-5,-4,-3,-2,-1,0,1,10,20,30,33,34,70]  Table=[-10,-10,0,1,2,3,4,5,6,7,8,9,10,33,33,33,33,33,33,33]  LookUpMeth=Use Input Nearest  OutDataTypeMode=single  OutDataType=fixdt(1, 16)  OutScaling=2^0  OutDataTypeStr=single  RndMeth=Nearest
  Terminator{,1,8..10} (5 alike) : Terminator
  Unit Delay : UnitDelay  SampleTime=-1
  Unit Delay1 : UnitDelay  SampleTime=-1
  wires:
  BatTemp/1 -> NewNameGeo/1, [BatTemp]  "MyBatTemp"
  ChillerOnOff/1 -> ChillerStateFlow/3(ChillerOnOff)
  ChillerT_SP/1 -> CreateChillerSPCmnd/1(ChillerT_SP)
  CreateChillerSPCmnd2/1(SetChillerSPCmnd) -> ChillerStateFlow/1(BatTempSwitchSlct)
  ChillerStateFlow/4(ReadChillerSP_Action) -> [ReadChillerSP_Action]
  ChillerOpMode/1 -> ChillerStateFlow/4(ChillerOpMode)
  CreateChillerSPCmnd/1(SetChillerSPCmnd) -> ChillerStateFlow/2(ManualChillerSP_Cmnd)
  ChillerStateFlow/1(ChillerTx) -> [ChillerTx]
  ChillerStateFlow/5(ReadChillerTemp_Action) -> [ReadChillerTemp_Action]
  ChillerStateFlow/2(ChillerTxNumBytes) -> [ChillerTxNumBytes]
  ChillerStateFlow/3(ChillerRxNumBytes) -> [ChillerRxNumBytes]
  DS2211SER_TX_B2/1 -> Gain3/1
  DS2211SER_TX_B2/2 -> Gain4/1
  DS2211SER_RX_B2/1 -> Gain/1
  DS2211SER_RX_B2/3 -> Gain2/1
  [ChillerTx] -> DS2211SER_TX_B2/1
  [ChillerTxNumBytes] -> DS2211SER_TX_B2/2
  [ChillerRxNumBytes] -> DS2211SER_RX_B2/1
  ChillerCommands/1(TurnChiller_On) -> [TurnChiller_On]
  ChillerCommands/2(TurnChiller_Off) -> [TurnChiller_Off]
  ChillerCommands/3(SetEcho_On) -> [SetEcho_On]
  ChillerCommands/4(ReadChiller_Status) -> [ReadChiller_Status]
  ChillerCommands/5(ReadChillerSetPoint) -> [ReadChillerSetPoint]
  ChillerCommands/6(ReadChiller_Temp) -> [ReadChiller_Temp]
  [TurnChiller_On] -> ChillerStateFlow/5(TurnChiller_On)
  [TurnChiller_Off] -> ChillerStateFlow/6(TurnChiller_Off)
  [ReadChillerSetPoint] -> ChillerStateFlow/7(ReadChillerSP)
  [ReadChiller_Temp] -> ChillerStateFlow/8(ReadChillerTemp)
  [PosResp] -> ChillerStateFlow/9(PositiveResponse)
  [SetEcho_On] -> Terminator1/1
  [ReadChiller_Status] -> ChillerStateFlow/10(ReadChillerStatus)
  [ChillerOn] -> ChillerStateFlow/11(ChillerOn)
  DS2211SER_RX_B2/2 -> Gain1/1
  [ChillerRxBytes] -> ChillerRxProcessing/1(RxBytes)
  [ChillerActRx] -> ChillerRxProcessing/2(NumRxBytes)
  ChillerStateFlow/6(ReadChillerStatus_Action) -> [ReadChillerStatus_Action]
  [ReadChillerStatus_Action] -> ChillerRxProcessing/4(ReadChillerStatus_Action)
  ChillerRxProcessing/1(ChillerPosResponse) -> Unit Delay/1
  ChillerRxProcessing/2(ChillerOn) -> Unit Delay1/1
  ManualChillerPower/1 -> ChillerStateFlow/12(ManualChillerPower)
  ChillerStateFlow/7(ChillerPowerStatus) -> Terminator/1
  Unit Delay/1 -> [PosResp]  "PosResp"
  Unit Delay1/1 -> [ChillerOn]  "ChillerOn"
  Gain/1 -> [ChillerRxBytes]  "ChillerRxBytes"
  Gain1/1 -> [ChillerActRx]  "ChillerActRx"
  Gain2/1 -> Terminator10/1  "ChillerRxStatus"
  Gain3/1 -> Terminator8/1  "ChillerTxBytes"
  Gain4/1 -> Terminator9/1  "ChillerTxStatus"
  ChillerStateFlow/8(WaitRx) -> [WaitRx]
  [WaitRx] -> ChillerRxProcessing/3(WaitRx)
  [ReadChillerTemp_Action] -> ChillerRxProcessing/6(ReadChillerTemp_Action)
  [ReadChillerSP_Action] -> ChillerRxProcessing/5(ReadChillerSP_Action)
  [BatTemp] -> ChillerStateFlow/13(BatTemp)
  NewNameGeo/1 -> Gain5/1
  Gain5/1 -> CreateChillerSPCmnd2/1(ChillerT_SP)  "BatTempAfterTable"

== system HIL_Testing_SW/TX/Chiller/Trigger_200ms1 ==
  Function-Call Generator : simulink/Ports & Subsystems/Function-Call Generator  sample_time=.3  numberOfIterations=1
  Output Parameter : Outport  OutDataType=sfix(16)  OutScaling=2^0
  wires:
  Function-Call Generator/1 -> Output Parameter/1
